simulink model "test_4"  (R2022a)
settings: Solver=ode4  StartTime=0.0  StopTime=50  FixedStep=0.01  RelTol=1e-3
libraries: simulink x1
settings Model: Creator=Alireza Sharifi  LastModifiedBy=Alireza Sharifi

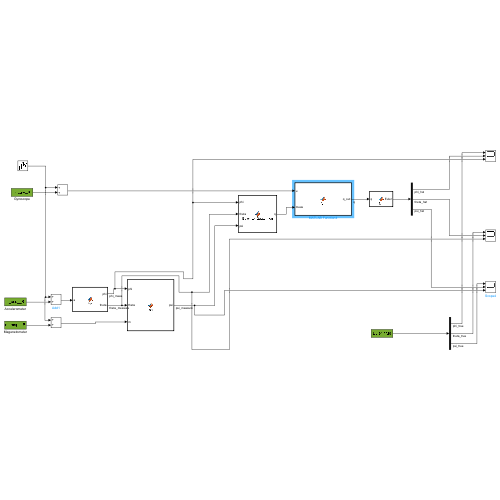
[thumbnail: Simulink's stored preview of the top-level diagram]
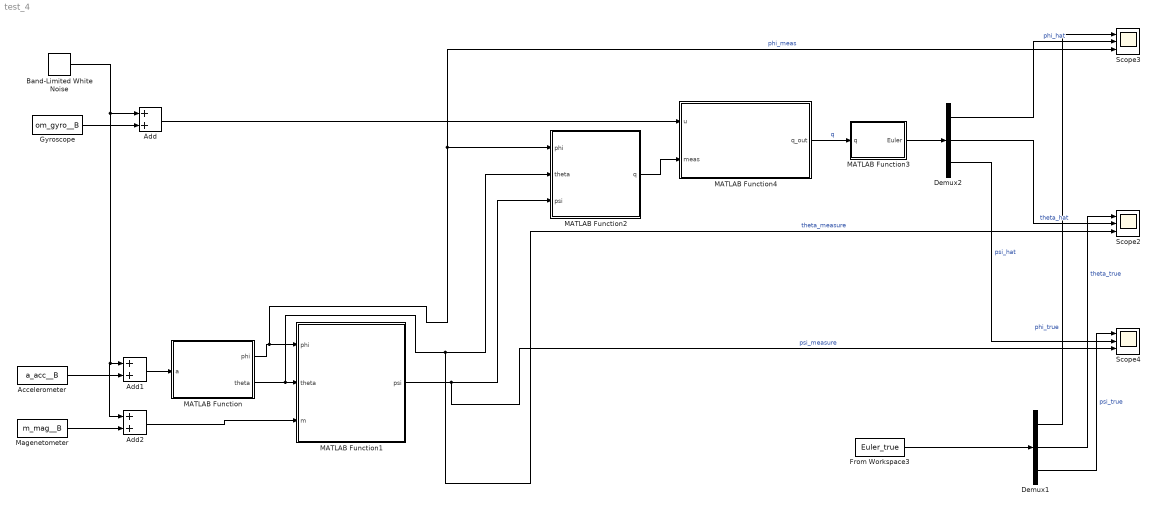
== system test_4 ==
  Accelerometer : FromWorkspace  VariableName=a_acc__B  SampleTime=0.01
  Add : Sum
  Add1 : Sum
  Add2 : Sum
  Band-Limited White Noise : simulink/Sources/Band-Limited White Noise  Cov=1e-5  Ts=0.01  seed=[23341]
  Demux1 : Demux  Outputs=3
  Demux2 : Demux  Outputs=3
  From Workspace3 : FromWorkspace  VariableName=Euler_true  SampleTime=0.01
  Gyroscope : FromWorkspace  VariableName=om_gyro__B  SampleTime=0.01
  MATLAB Function : MATLAB Function  TreatAsAtomicUnit=on
  MATLAB Function1 : MATLAB Function  TreatAsAtomicUnit=on
  MATLAB Function2 : MATLAB Function  TreatAsAtomicUnit=on
  MATLAB Function3 : MATLAB Function  TreatAsAtomicUnit=on
  MATLAB Function4 : MATLAB Function  TreatAsAtomicUnit=on
  Magenetometer : FromWorkspace  VariableName=m_mag__B  SampleTime=0.01
  Scope2 : Scope  NumInputPorts=3
  Scope3 : Scope  NumInputPorts=3
  Scope4 : Scope  NumInputPorts=3
  wires:
  Gyroscope/1 -> Add/2
  Add/1 -> MATLAB Function4/1(u)
  Accelerometer/1 -> Add1/2
  Magenetometer/1 -> Add2/2
  Band-Limited White Noise/1 -> Add/1, Add2/1, Add1/1
  From Workspace3/1 -> Demux1/1
  MATLAB Function4/1(q_out) -> MATLAB Function3/1(q)  "q"
  MATLAB Function2/1(q) -> MATLAB Function4/2(meas)
  MATLAB Function/2(theta) -> MATLAB Function2/2(theta), Scope2/3, MATLAB Function1/2(theta)  "theta_measure"
  Add1/1 -> MATLAB Function/1(a)
  Add2/1 -> MATLAB Function1/3(m)
  MATLAB Function/1(phi) -> MATLAB Function2/1(phi), Scope3/3, MATLAB Function1/1(phi)  "phi_meas"
  MATLAB Function1/1(psi) -> MATLAB Function2/3(psi), Scope4/3  "psi_measure"
  MATLAB Function3/1(Euler) -> Demux2/1
  Demux2/1 -> Scope3/2  "phi_hat"
  Demux2/2 -> Scope2/2  "theta_hat"
  Demux2/3 -> Scope4/2  "psi_hat"
  Demux1/1 -> Scope3/1  "phi_true"
  Demux1/2 -> Scope2/1  "theta_true"
  Demux1/3 -> Scope4/1  "psi_true"

== matlab function test_4/MATLAB Function1 ==
  data: phi input; psi output; theta input; m input
function psi = fcn(phi,theta,m)
mx=m(1);
my=m(2);
mz=m(3);
%
num_psi=-cos(phi)*my+sin(phi)*mz;
den_psi=cos(theta)*mx+sin(theta)*sin(phi)*my+sin(theta)*cos(phi)*mz;
declination_angle=-4.0266*pi/180;
psi=atan2(num_psi,den_psi)+declination_angle;

== matlab function test_4/MATLAB Function ==
  data: a input; phi output; theta output
function [phi,theta] = fcn(a)
ax=a(1);
ay=a(2);
az=a(3);
g=9.81;
phi=atan2(-ay,-az);
theta=asin(ax/g);

== matlab function test_4/MATLAB Function2 ==
  data: phi input; q output; theta input; psi input
function q = Euler_to_Quaternion(phi,theta,psi)

q0 = cos(psi/2)*cos(theta/2)*cos(phi/2) + sin(psi/2)*sin(theta/2)*sin(phi/2);
q1 = cos(psi/2)*cos(theta/2)*sin(phi/2) - sin(psi/2)*sin(theta/2)*cos(phi/2);
q2 = cos(psi/2)*sin(theta/2)*cos(phi/2) + sin(psi/2)*cos(theta/2)*sin(phi/2);
q3 = sin(psi/2)*cos(theta/2)*cos(phi/2) - cos(psi/2)*sin(theta/2)*sin(phi/2);

q = [q0, q1, q2, q3];

end

== matlab function test_4/MATLAB Function3 ==
  data: q input; Euler output
function Euler = fcn(q)

q0 = q(1);
q1 = q(2);
q2 = q(3);
q3 = q(4);

phi = atan2(2*(q0*q1 + q2*q3), (q0^2 + q3^2 - q1^2 - q2^2));
theta = asin(2*(q0*q2 - q1*q3));
psi = atan2(2*(q0*q3 + q1*q2), (q0^2 + q1^2 - q2^2 - q3^2));

Euler = [phi, theta, psi];

end

== matlab function test_4/MATLAB Function4 ==
  data: u input; q_out output; meas input
function q_out = fcn(u, meas)

q0 = meas(1);
q1 = meas(2);
q2 = meas(3);
q3 = meas(4);

p = u(1);
q = u(2);
r = u(3);

y_m = [q0; q1; q2; q3];

Ts = 0.01;
    
    Q = 1e-4*[1 0 0 0
              0 1 0 0
              0 0 1 0
              0 0 0 1];

    R = 1e-2*[1 0 0 0
              0 1 0 0
              0 0 1 0
              0 0 0 1];

    persistent q_hat P
    
    if isempty(q_hat)
        q_hat = 0*[q0; q1; q2; q3];
    end
    if isempty(P)
        P=[100 0 0 0
            0 100 0 0
            0 0 100 0
            0 0 0 100];
    end
%%
    q_hat = q_hat + 0.5*Ts*[0 -p -q -r; p 0 r -q; q -r 0 p; r q -p 0]*q_hat;
    %%
    A = 0.5*Ts*[0 -p -q -r; p 0 r -q; q -r 0 p; r q -p 0];
    F = eye(4) + A;
    P = F*P*F'+ Q;
    %%
    y_hat = q_hat;
    C = eye(4);
    K = P*C'*inv(C*P*C' + R);
    q_hat = q_hat + K*(y_m - y_hat);
    P = (eye(4) - K*C)*P*(eye(4) - K*C)' + K*R*K';
    q_out = q_hat;
end
